simulink model "teste_motor_v10"  (R2025b)
settings: Solver=VariableStepAuto  StartTime=0.0  StopTime=10  RelTol=1e-3
undefined symbols (not defined in the file): fdesignblkfcn, gcbh, Kad, Kre
libraries: nesl_utility x26, fl_lib x25, simulink x19, dsparch4 x3, sdl_lib x2, simulink_extras x2, dspfdesign x1
(part 3 of 3)

== system teste_motor_v10/Motor de Sem Controle/Subsystem2/Subsystem1/Medições/Filtro/Subsystem2/Subsystem ==
  Rel Spark : Inport
  RPM : Inport  Port=2
  2-D Lookup Table : Lookup_n-D  BreakpointsForDimension1=[15, 18, 20, 25, 30]  BreakpointsForDimension2=[800, 1000, 1500, 1800, 2000]  Table=[0 0 0 0 0; 0.05 0.05 0.02 0.01 0.01; 0.2 0.15 0.1 0.05 0.05; 0.6 0.5 0.3 0.2 0.1; 0.95 0.9 0.8 0.6 0.4]  InternalRulePriority=Speed  RndMeth=Simplest
      settings: InputPortMap=u0,u1
  Constant4 : Constant
  Relational Operator : RelationalOperator  Operator=<  OutDataTypeStr=boolean  RndMeth=Simplest  InputSameDT=off
  Subtract : Sum  Inputs=+-
  Uniform Random Number : UniformRandomNumber  Minimum=0  SampleTime=0.1
  Unit Delay : UnitDelay  SampleTime=-1  HasFrameUpgradeWarning=on
  knock : Outport
  wires:
  2-D Lookup Table/1 -> Subtract/2
  RPM/1 -> 2-D Lookup Table/2
  Relational Operator/1 -> Unit Delay/1
  Unit Delay/1 -> knock/1
  Rel Spark/1 -> 2-D Lookup Table/1
  Uniform Random Number/1 -> Relational Operator/2
  Subtract/1 -> Relational Operator/1
  Constant4/1 -> Subtract/1

== system teste_motor_v10/Motor de Sem Controle/Subsystem2/Subsystem1/Medições/Sensor/Subsystem4/Subsystem ==
  u : Inport
  AND : Logic  Inputs=3  IconShape=distinctive  AllPortsSameDT=off  OutDataTypeStr=boolean
  Compare To Constant : simulink/Logic and Bit Operations/Compare To Constant  relop=>  const=0  OutDataTypeStr=boolean
  Compare To Constant1 : simulink/Logic and Bit Operations/Compare To Constant  relop=>  const=0  OutDataTypeStr=boolean
  NOT : Logic  Operator=NOT  IconShape=distinctive  AllPortsSameDT=off  OutDataTypeStr=boolean
  Unit Delay : UnitDelay  SampleTime=-1  HasFrameUpgradeWarning=on
  Borda de Subida : Outport
  wires:
  u/1 -> Compare To Constant1/1, AND/2, Compare To Constant/1
  Unit Delay/1 -> NOT/1
  AND/1 -> Borda de Subida/1
  NOT/1 -> AND/1
  Compare To Constant/1 -> Unit Delay/1
  Compare To Constant1/1 -> AND/3

== system teste_motor_v10/Motor de Sem Controle/Subsystem2/Subsystem1/Medições/Sensor/Subsystem4/Subsystem1 ==
  u : Inport
  Compare To Constant : simulink/Logic and Bit Operations/Compare To Constant  relop===  const=0  OutDataTypeStr=boolean
  Constant : Constant
  Constant1 : Constant  Value=0
  Sum : Sum
  Switch : Switch  Criteria=u2 > Threshold  SaturateOnIntegerOverflow=off  InputSameDT=off
  Unit Delay : UnitDelay  SampleTime=-1  HasFrameUpgradeWarning=on
  Contagem : Outport
  wires:
  Compare To Constant/1 -> Switch/2
  Unit Delay/1 -> Contagem/1, Sum/1
  Constant1/1 -> Switch/3
  Sum/1 -> Switch/1
  Switch/1 -> Unit Delay/1
  u/1 -> Compare To Constant/1
  Constant/1 -> Sum/2

== system teste_motor_v10/Motor de Sem Controle/Subsystem2/Subsystem1/Medições/Sensor/Subsystem4/Subsystem3 ==
  In1 : Inport
  u : Inport  Port=2
  In3 : Inport  Port=3
  AND : Logic  IconShape=distinctive  AllPortsSameDT=off  OutDataTypeStr=boolean
  Compare To Constant : simulink/Logic and Bit Operations/Compare To Constant  relop=>=  const=5000  OutDataTypeStr=boolean
  Constant : Constant  Value=0
  Switch : Switch  Criteria=u2 > Threshold  SaturateOnIntegerOverflow=off  InputSameDT=off
  Out1 : Outport
  wires:
  u/1 -> Compare To Constant/1
  In1/1 -> Switch/1
  AND/1 -> Switch/2
  Compare To Constant/1 -> AND/1
  Constant/1 -> Switch/3
  Switch/1 -> Out1/1
  In3/1 -> AND/2

== matlab function teste_motor_v10/Motor de Sem Controle/Knock Control1/bypass ==
  settings: updateMethod=DISCRETE
  data: knock input; bypass_mode output; pos input
function bypass_mode = monitor_de_knock(knock, pos)
% Variáveis que guardam memória
persistent knock_count teve_knock_no_ciclo ultima_posicao trava_seguranca

% Inicialização
if isempty(knock_count)
    knock_count = 0;
    teve_knock_no_ciclo = 0;
    ultima_posicao = 0;
    trava_seguranca = 0; % 0 = Normal, 1 = Travado em Bypass
end

% Se a trava já foi acionada, mantém o output em 2 para sempre
if trava_seguranca == 1
    bypass_mode = 2;
    return; % Sai da função aqui, ignorando o resto
end

% --- Lógica de Contagem (só roda se não estiver travado) ---

% 1. Detecta batida no ciclo atual
if knock > 0.5 
    teve_knock_no_ciclo = 1;
end

% 2. Verifica fim do ciclo (720 -> 0 graus)
if pos < (ultima_posicao - 100)
    if teve_knock_no_ciclo == 1
        knock_count = knock_count + 1;
    else
        knock_count = 0; % Reset se o ciclo foi limpo
    end
    teve_knock_no_ciclo = 0; 
end

ultima_posicao = pos;

% 3. Verificação do Gatilho
if knock_count >= 20
    trava_seguranca = 1; % Ativa a trava permanentemente
    bypass_mode = 2;
else
    bypass_mode = 1;
end

== matlab function teste_motor_v10/Motor de Sem Controle/Subsystem/Leituras/Knock/MATLAB Function ==
  data: rpm input; knock_probabilidade output; AFR input; SA input
function knock_probabilidade = fcn(rpm, AFR, SA)

    rpm_limite_min = 1000;
    SA_limite_min = 3;
    AFR_estq = 14.7;
    
    fator_rpm = max(0, (rpm - rpm_limite_min)/rpm_limite_min);
    fator_SA = max(0,(SA - SA_limite_min)/SA_limite_min);
    fator_AFR = AFR / AFR_estq;
    
    knock_probabilidade = (fator_rpm * fator_SA * fator_AFR^3)*200 + 1800;
end

== matlab function teste_motor_v10/Motor de Sem Controle/Knock Control1/Subsystem/MATLAB Function2 ==
  settings: updateMethod=DISCRETE
  data: u input; y output
function y = fcn(u)
    % u é a posição atual (0 a 720)
    
    % Declaramos 'ciclos' como persistente para ele manter o valor
    % entre um passo de simulação e outro.
    persistent ciclos pos_anterior
    
    % Inicialização na primeira vez que o modelo roda
    if isempty(ciclos)
        ciclos = 0;
        pos_anterior = 0;
    end
    
    % Lógica: se a posição atual caiu drasticamente (ex: de 719 para 2),
    % detectamos a virada do ciclo.
    if u < pos_anterior
        ciclos = ciclos + 1;
    end
    
    % Atualiza a memória para o próximo passo
    pos_anterior = u;
    
    % Saída do bloco
    y = ciclos;
end

== matlab function teste_motor_v10/Motor de Sem Controle/Knock Control1/Subsystem/MATLAB Function3 ==
  settings: updateMethod=DISCRETE
  data: amp input; is_knocking input; pos input; cicles_recover input; retard output; lock_out output; c_out output; ret_max input; ret_min input; amp_min input; lim_retard input
function [retard, lock_out, c_out] = knock_control(amp, is_knocking, pos, cicles_recover, ret_max, ret_min, amp_min, lim_retard)
    % =====================================================================
    % ESTRATÉGIA DE CONTROLE DE DETONAÇÃO (LOGARÍTMICA NÃO CONVENCIONAL)
    % =====================================================================
    % retard  : Valor de atraso de ignição (graus)
    % lock_out: Status da trava de segurança (1 = travado, 0 = liberado)
    % c_out   : Contador de ciclos desde o último evento de knock
    % =====================================================================

    persistent deg last_state lock c last_pos angulo_acumulado deg_no_knock targets teste
    
    % Inicialização das Variáveis Persistentes
    if isempty(deg)
        deg = 0;
        last_state = 0.0;
        lock = 1; 
        c = 1;
        last_pos = 0;
        angulo_acumulado = 0;
        deg_no_knock = 0;
        targets = [0];
        teste = 0;
    end
    
    % Converte is_knocking para número caso venha como lógico/booleano
    is_knocking_num = double(is_knocking);

    % CÁLCULO DO DESLOCAMENTO ANGULAR (Delta de graus)
    % Identifica quanto o motor girou entre as chamadas da função
    delta_pos = pos - last_pos;
    if delta_pos < 0 % Tratamento para o reset do ciclo (720 -> 0)
        delta_pos = delta_pos + 720;
        teste = 0;
    end

    % LÓGICA DE DETECÇÃO DE KNOCK (Atraso Imediato)
    if is_knocking_num > 0 && teste == 0
        if last_state == 0        % Detecta apenas a borda de subida do erro
            if deg < lim_retard           % Só adiciona checkpoints se o valor não for o máximo
                targets = [deg, targets];
            end
            % Calculamos o quanto a amplitude atual excedeu o mínimo
            excesso = amp - amp_min;
            % Criamos um fator de 0 a 1
            fator = excesso / (3*amp_min); 
            % Calculamos o degrau linear entre ret_min e ret_max
            degrau = ret_min + (fator * (ret_max - ret_min));
            % Aplica as travas: não pode ser menor que ret_min nem maior que ret_max
            degrau_final = max(ret_min, min(ret_max, degrau));
            deg = deg + degrau_final;
            %deg = deg + max(0.5, ((5*amp - 71) / 18));      % Degrau de retardo
            deg = min(deg, lim_retard);   % Saturação de segurança (retardo máximo)
            c = 1;                % Reseta contador de ciclos
            deg_no_knock = deg;   % Armazena referência para a curva
            teste = 1;
        end
        lock = 1;                 % Ativa trava de segurança
        angulo_acumulado = 0;     % Reseta contagem de espera
    end

    % LIBERAÇÃO DINÂMICA (Janela de Segurança)
    % Garante que o motor gire uma quantidade mínima de graus em silêncio antes de recuperar
    if lock == 1 && is_knocking_num == 0
        angulo_acumulado = angulo_acumulado + delta_pos;
        
        if angulo_acumulado > 800 % Define a distância segura entre janelas
            lock = 0; 
            angulo_acumulado = 0;
        end
    end

    % RECUPERAÇÃO E CONTADOR DE CICLOS (Estratégia não convencional)
    % Parâmetros baseados em probabilidade estatística Pref = 0.01 (1%)
    % Pref = 0.01;
    % Nref = 1/Pref; % Alvo de 100 ciclos para zerar o retardo
    
    if lock == 0 && is_knocking_num == 0
        % A recuperação ocorre apenas uma vez por ciclo completo do motor
        if targets(1) >= (lim_retard - 0.01)
            targets(1) = [];
        end

        if pos < last_pos
            c = c + 1;

            % Cálculo do progresso logarítmico normalizado
            % Garante suavidade e precisão de retorno em Nref ciclos
            current_target = targets(1);
            progresso = log(min(c, cicles_recover)) / log(cicles_recover);
            deg = deg_no_knock - (progresso * (deg_no_knock - current_target));
            if c >= cicles_recover
                % Se ainda não chegamos no zero absoluto, 'limpamos' o patamar alcançado
                % e iniciamos a descida para o próximo valor do vetor
                if numel(targets)>1
                    deg = targets(1);
                    deg_no_knock = deg;
                    targets(1) = []; % Deleta o primeiro elemento, o vetor "encolhe"
                    c = 1;
                else
                    deg = 0;
                end
            end
        end
    end
    % ATUALIZAÇÃO DE ESTADOS E SATURAÇÃO FINAL
    last_pos = pos;
    last_state = is_knocking_num;
    
    % Garante que o valor final esteja dentro dos limites operacionais [0, 15]
    deg = max(0, min(deg, lim_retard));
    
    % Saídas do bloco
    retard = deg;
    lock_out = lock;
    c_out = c;

end
